simulink model "chybam3a"  (R2021b)
settings: Solver=ode45  StartTime=0.0  StopTime=15  MaxStep=0.01  RelTol=1e-3
settings Model: Creator=Student  LastModifiedBy=Student

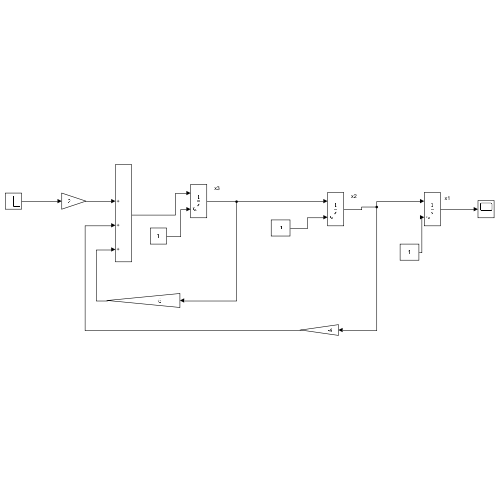
[thumbnail: Simulink's stored preview of the top-level diagram]
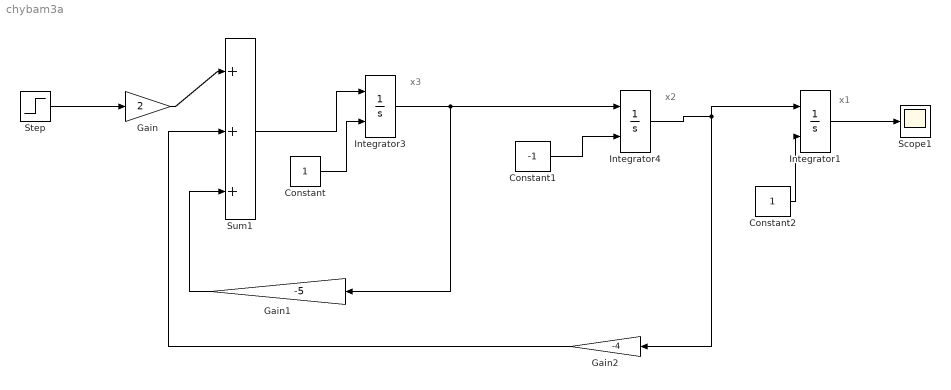
== system chybam3a ==
  note: x3
  note: x2
  note: x1
  Constant : Constant
  Constant1 : Constant  Value=-1
  Constant2 : Constant
  Gain : Gain  Gain=2
  Gain1 : Gain  Gain=-5
  Gain2 : Gain  Gain=-4
  Integrator1 : Integrator  InitialConditionSource=external
  Integrator3 : Integrator  InitialConditionSource=external
  Integrator4 : Integrator  InitialConditionSource=external
  Scope1 : Scope
  Step : Step  Time=0.01  Before=100  After=0  SampleTime=0
  Sum1 : Sum  Inputs=|+++
  wires:
  Integrator3/1 -> Gain1/1, Integrator4/1
  Gain/1 -> Sum1/1
  Constant1/1 -> Integrator4/2
  Integrator4/1 -> Gain2/1, Integrator1/1
  Sum1/1 -> Integrator3/1
  Constant/1 -> Integrator3/2
  Gain1/1 -> Sum1/3
  Gain2/1 -> Sum1/2
  Constant2/1 -> Integrator1/2
  Integrator1/1 -> Scope1/1
  Step/1 -> Gain/1
